simulink model "simulador4"  (Simulink 2.09)
settings: Solver=ode4  StartTime=0.0  StopTime=1  FixedStep=1e-4  MaxStep=0.1  RelTol=1e-3  AbsTol=1e-3
settings Model: SaveTime=off  SaveOutput=off  ConsistencyChecking=off  RTWTemplateMakefile=grt_vc.tmf

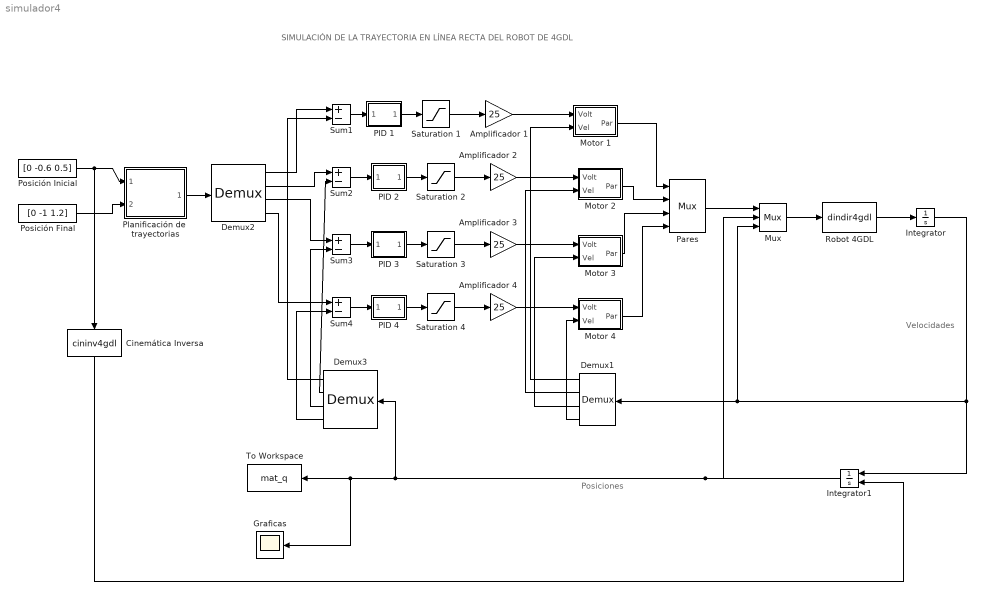
== system simulador4 ==
  note: Velocidades
  note: Posiciones
  note: SIMULACIÓN DE LA TRAYECTORIA EN LÍNEA RECTA DEL ROBOT DE 4GDL
  Amplificador {1..4} (4 alike) : Gain  Gain=25
  Cinemática Inversa : MATLABFcn  Orientation=down  MATLABFcn=cininv4gdl  OutputWidth=4
  Demux1 : Demux  Orientation=left  Outputs=4
  Demux2 : Demux  Outputs=4
  Demux3 : Demux  Orientation=left  Outputs=4
  Graficas : Scope
      settings: TickLabels=on  TimeRange=auto  YMin=-3.25  YMax=1  SaveToWorkspace=off  SaveName=ScopeData
  Integrator : Integrator  ExternalReset=none  InitialConditionSource=internal  InitialCondition=[0 0 0 0]  LimitOutput=off  UpperSaturationLimit=inf  LowerSaturationLimit=-inf  ShowSaturationPort=off  ShowStatePort=off  AbsoluteTolerance=auto
  Integrator1 : Integrator  Orientation=left  ExternalReset=none  InitialConditionSource=external  InitialCondition=[0 0 0 0]  LimitOutput=off  UpperSaturationLimit=inf  LowerSaturationLimit=-inf  ShowSaturationPort=off  ShowStatePort=off  AbsoluteTolerance=auto
  Motor 1 : Subsystem  mask(Motor){R=0.39, L=0.00065, Kt=0.054, Kv=0.054, imax=25.3, red=500}
      mask prompts: R "Resistencia (Ohmios)"; L "Inductancia (Henrios)"; Kt "Kt (Nm/A)"; Kv "Kv (V/rad/s)"; imax "Corriente máxima (Amperios)"; red "Reductor"
  Motor 2 : Subsystem  mask(Motor){R=1.6, L=0.00156, Kt=0.176, Kv=0.176, imax=23.7, red=2}
      mask prompts: R "Resistencia (Ohmios)"; L "Inductancia (Henrios)"; Kt "Kt (Nm/A)"; Kv "Kv (V/rad/s)"; imax "Corriente máxima (Amperios)"; red "Reductor"
  Motor 3 : Subsystem  mask(Motor){R=0.8, L=0.00093, Kt=0.058, Kv=0.058, imax=18.5, red=2}
      mask prompts: R "Resistencia (Ohmios)"; L "Inductancia (Henrios)"; Kt "Kt (N-m)"; Kv "Kv (V/rad/s)"; imax "Corriente máxima (Amperios)"; red "Reductor"
  Motor 4 : Subsystem  mask(Motor){R=6.9, L=0.00128, Kt=0.035, Kv=0.035, imax=3.6, red=500}
      mask prompts: R "Resistencia (Ohmios)"; L "Inductancia (Henrios)"; Kt "Kt (N-m)"; Kv "Kv (V/rad/s)"; imax "Corriente máxima (Amperios)"; red "Reductor"
  Mux : Mux  Inputs=3
  PID 1 : Subsystem  mask(PID Controller){P=90, I=0, D=1.6}
      mask prompts: P "Proportional:"; I "Integral"; D "Derivative:"
      mask help:
      | Enter expressions for proportional, integral, and derivative terms.
      | P+I/s+Ds
      mask Help: This block implements a PID controller where parameters are entered for the Proportional, Integral and Derivative terms. Unmask this block to see how it works. The derivative term is implemented using a true derivative block.
      mask Display: disp('PID')
  PID 2 : Subsystem  mask(PID Controller){P=300, I=0, D=6}
      mask prompts: P "Proportional:"; I "Integral"; D "Derivative:"
      mask help:
      | Enter expressions for proportional, integral, and derivative terms.
      | P+I/s+Ds
      mask Help: This block implements a PID controller where parameters are entered for the Proportional, Integral and Derivative terms. Unmask this block to see how it works. The derivative term is implemented using a true derivative block.
      mask Display: disp('PID')
  PID 3 : Subsystem  mask(PID Controller){P=200, I=0, D=5.7}
      mask prompts: P "Proportional:"; I "Integral"; D "Derivative:"
      mask help:
      | Enter expressions for proportional, integral, and derivative terms.
      | P+I/s+Ds
      mask Help: This block implements a PID controller where parameters are entered for the Proportional, Integral and Derivative terms. Unmask this block to see how it works. The derivative term is implemented using a true derivative block.
      mask Display: disp('PID')
  PID 4 : Subsystem  mask(PID Controller){P=100, I=0, D=0}
      mask prompts: P "Proportional:"; I "Integral"; D "Derivative:"
      mask help:
      | Enter expressions for proportional, integral, and derivative terms.
      | P+I/s+Ds
      mask Help: This block implements a PID controller where parameters are entered for the Proportional, Integral and Derivative terms. Unmask this block to see how it works. The derivative term is implemented using a true derivative block.
      mask Display: disp('PID')
  Pares : Mux  Inputs=4
  Planificación de  trayectorias : Subsystem
      mask Type: Planificación de trayectorias
      mask Display: disp('Planificación')
  Posición Final : Constant  Value=[0 -1 1.2]
  Posición Inicial : Constant  Value=[0 -0.6 0.5]
  Robot 4GDL : MATLABFcn  MATLABFcn=dindir4gdl  OutputWidth=4
  Saturation {1..4} (4 alike) : Saturate  UpperLimit=10  LowerLimit=-10
  Sum{1..4} (4 alike) : Sum  Inputs=+-
  To Workspace : ToWorkspace  VariableName=mat_q  SampleTime=-1
  wires:
  Planificación de  trayectorias/1(Posiciones Articulares) -> Demux2/1
  Cinemática Inversa/1 -> Integrator1/2
  Posición Inicial/1 -> Cinemática Inversa/1, Planificación de  trayectorias/1(Posición Inicial)
  Posición Final/1 -> Planificación de  trayectorias/2(Posición Final)
  Integrator1/1 -> Graficas/1, To Workspace/1, Demux3/1, Mux/2
  Amplificador 3/1 -> Motor 3/1(Volt)
  Amplificador 2/1 -> Motor 2/1(Volt)
  Demux1/2 -> Motor 2/2(Vel)
  Motor 3/1(Par) -> Pares/3
  Motor 2/1(Par) -> Pares/2
  Motor 1/1(Par) -> Pares/1
  Demux1/1 -> Motor 1/2(Vel)
  Demux1/3 -> Motor 3/2(Vel)
  Amplificador 1/1 -> Motor 1/1(Volt)
  Mux/1 -> Robot 4GDL/1
  Pares/1 -> Mux/1
  Demux2/1 -> Sum1/1
  Demux2/2 -> Sum2/1
  Demux2/3 -> Sum3/1
  Demux3/1 -> Sum1/2
  Demux3/2 -> Sum2/2
  Demux3/3 -> Sum3/2
  Sum2/1 -> PID 2/1(In_1)
  Sum3/1 -> PID 3/1(In_1)
  Sum1/1 -> PID 1/1(In_1)
  PID 1/1(Out_1) -> Saturation 1/1
  Saturation 1/1 -> Amplificador 1/1
  PID 2/1(Out_1) -> Saturation 2/1
  Saturation 2/1 -> Amplificador 2/1
  PID 3/1(Out_1) -> Saturation 3/1
  Saturation 3/1 -> Amplificador 3/1
  Integrator/1 -> Integrator1/1, Demux1/1, Mux/3
  Robot 4GDL/1 -> Integrator/1
  Amplificador 4/1 -> Motor 4/1(Volt)
  Sum4/1 -> PID 4/1(In_1)
  PID 4/1(Out_1) -> Saturation 4/1
  Saturation 4/1 -> Amplificador 4/1
  Demux1/4 -> Motor 4/2(Vel)
  Motor 4/1(Par) -> Pares/4
  Demux2/4 -> Sum4/1
  Demux3/4 -> Sum4/2

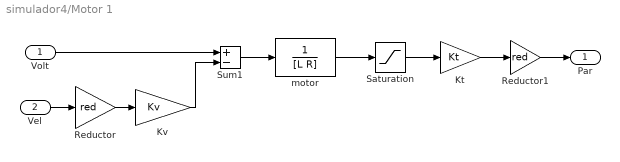
== system simulador4/Motor 1 ==
  Volt : Inport  Port=1  PortWidth=-1  SampleTime=-1
  Vel : Inport  Port=2  PortWidth=-1  SampleTime=-1
  Kt : Gain  Gain=Kt
  Kv : Gain  Gain=Kv
  Reductor : Gain  Gain=red
  Reductor1 : Gain  Gain=red
  Saturation : Saturate  UpperLimit=imax  LowerLimit=-imax
  Sum1 : Sum  Inputs=+-
  motor : TransferFcn  Numerator=[1]  Denominator=[L R]
  Par : Outport  Port=1  InitialOutput=0
  wires:
  Saturation/1 -> Kt/1
  motor/1 -> Saturation/1
  Kt/1 -> Reductor1/1
  Reductor1/1 -> Par/1
  Sum1/1 -> motor/1
  Reductor/1 -> Kv/1
  Kv/1 -> Sum1/2
  Volt/1 -> Sum1/1
  Vel/1 -> Reductor/1

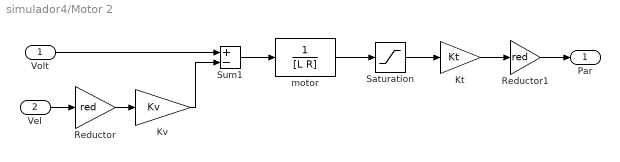
== system simulador4/Motor 2 ==
  Volt : Inport  Port=1  PortWidth=-1  SampleTime=-1
  Vel : Inport  Port=2  PortWidth=-1  SampleTime=-1
  Kt : Gain  Gain=Kt
  Kv : Gain  Gain=Kv
  Reductor : Gain  Gain=red
  Reductor1 : Gain  Gain=red
  Saturation : Saturate  UpperLimit=imax  LowerLimit=-imax
  Sum1 : Sum  Inputs=+-
  motor : TransferFcn  Numerator=[1]  Denominator=[L R]
  Par : Outport  Port=1  InitialOutput=0
  wires:
  Vel/1 -> Reductor/1
  Volt/1 -> Sum1/1
  Kv/1 -> Sum1/2
  Reductor/1 -> Kv/1
  Sum1/1 -> motor/1
  Reductor1/1 -> Par/1
  Kt/1 -> Reductor1/1
  motor/1 -> Saturation/1
  Saturation/1 -> Kt/1

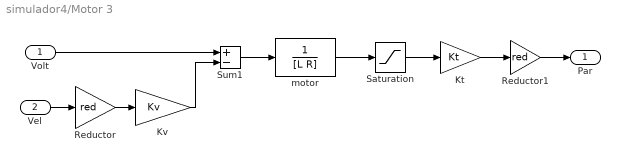
== system simulador4/Motor 3 ==
  Volt : Inport  Port=1  PortWidth=-1  SampleTime=-1
  Vel : Inport  Port=2  PortWidth=-1  SampleTime=-1
  Kt : Gain  Gain=Kt
  Kv : Gain  Gain=Kv
  Reductor : Gain  Gain=red
  Reductor1 : Gain  Gain=red
  Saturation : Saturate  UpperLimit=imax  LowerLimit=-imax
  Sum1 : Sum  Inputs=+-
  motor : TransferFcn  Numerator=[1]  Denominator=[L R]
  Par : Outport  Port=1  InitialOutput=0
  wires:
  Saturation/1 -> Kt/1
  motor/1 -> Saturation/1
  Kt/1 -> Reductor1/1
  Reductor1/1 -> Par/1
  Sum1/1 -> motor/1
  Reductor/1 -> Kv/1
  Kv/1 -> Sum1/2
  Volt/1 -> Sum1/1
  Vel/1 -> Reductor/1

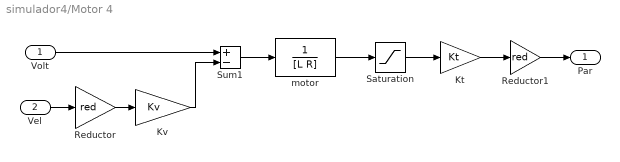
== system simulador4/Motor 4 ==
  Volt : Inport  Port=1  PortWidth=-1  SampleTime=-1
  Vel : Inport  Port=2  PortWidth=-1  SampleTime=-1
  Kt : Gain  Gain=Kt
  Kv : Gain  Gain=Kv
  Reductor : Gain  Gain=red
  Reductor1 : Gain  Gain=red
  Saturation : Saturate  UpperLimit=imax  LowerLimit=-imax
  Sum1 : Sum  Inputs=+-
  motor : TransferFcn  Numerator=[1]  Denominator=[L R]
  Par : Outport  Port=1  InitialOutput=0
  wires:
  Vel/1 -> Reductor/1
  Volt/1 -> Sum1/1
  Kv/1 -> Sum1/2
  Reductor/1 -> Kv/1
  Sum1/1 -> motor/1
  Reductor1/1 -> Par/1
  Kt/1 -> Reductor1/1
  motor/1 -> Saturation/1
  Saturation/1 -> Kt/1

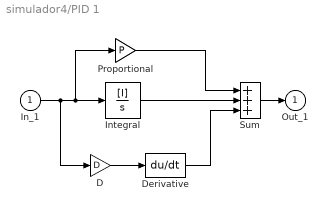
== system simulador4/PID 1 ==
  In_1 : Inport  Port=1  PortWidth=-1  SampleTime=-1
  D : Gain  Gain=D
  Derivative : Derivative
  Integral : TransferFcn  Numerator=[I]  Denominator=[1 0]
  Proportional : Gain  Gain=P
  Sum : Sum  Inputs=+++
  Out_1 : Outport  Port=1  InitialOutput=0
  wires:
  Proportional/1 -> Sum/1
  Integral/1 -> Sum/2
  Derivative/1 -> Sum/3
  In_1/1 -> Proportional/1, Integral/1, D/1
  Sum/1 -> Out_1/1
  D/1 -> Derivative/1

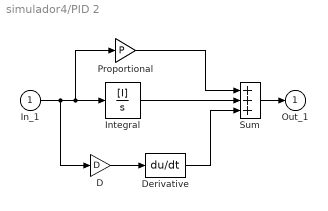
== system simulador4/PID 2 ==
  In_1 : Inport  Port=1  PortWidth=-1  SampleTime=-1
  D : Gain  Gain=D
  Derivative : Derivative
  Integral : TransferFcn  Numerator=[I]  Denominator=[1 0]
  Proportional : Gain  Gain=P
  Sum : Sum  Inputs=+++
  Out_1 : Outport  Port=1  InitialOutput=0
  wires:
  Proportional/1 -> Sum/1
  Integral/1 -> Sum/2
  Derivative/1 -> Sum/3
  In_1/1 -> Proportional/1, Integral/1, D/1
  Sum/1 -> Out_1/1
  D/1 -> Derivative/1

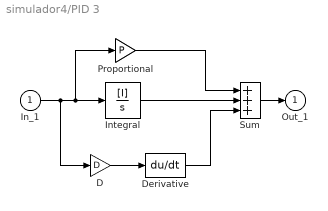
== system simulador4/PID 3 ==
  In_1 : Inport  Port=1  PortWidth=-1  SampleTime=-1
  D : Gain  Gain=D
  Derivative : Derivative
  Integral : TransferFcn  Numerator=[I]  Denominator=[1 0]
  Proportional : Gain  Gain=P
  Sum : Sum  Inputs=+++
  Out_1 : Outport  Port=1  InitialOutput=0
  wires:
  Proportional/1 -> Sum/1
  Integral/1 -> Sum/2
  Derivative/1 -> Sum/3
  In_1/1 -> Proportional/1, Integral/1, D/1
  Sum/1 -> Out_1/1
  D/1 -> Derivative/1

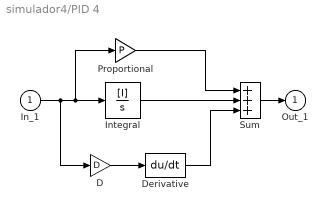
== system simulador4/PID 4 ==
  In_1 : Inport  Port=1  PortWidth=-1  SampleTime=-1
  D : Gain  Gain=D
  Derivative : Derivative
  Integral : TransferFcn  Numerator=[I]  Denominator=[1 0]
  Proportional : Gain  Gain=P
  Sum : Sum  Inputs=+++
  Out_1 : Outport  Port=1  InitialOutput=0
  wires:
  D/1 -> Derivative/1
  Sum/1 -> Out_1/1
  In_1/1 -> D/1, Integral/1, Proportional/1
  Derivative/1 -> Sum/3
  Integral/1 -> Sum/2
  Proportional/1 -> Sum/1

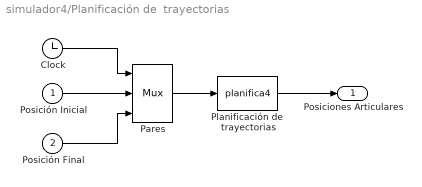
== system simulador4/Planificación de  trayectorias ==
  Posición Inicial : Inport  Port=1  PortWidth=-1  SampleTime=-1
  Posición Final : Inport  Port=2  PortWidth=-1  SampleTime=-1
  Clock : Clock
  Pares : Mux  Inputs=3
  Planificación de  trayectorias : MATLABFcn  MATLABFcn=planifica4  OutputWidth=4
  Posiciones Articulares : Outport  Port=1  InitialOutput=0
  wires:
  Clock/1 -> Pares/1
  Posición Inicial/1 -> Pares/2
  Posición Final/1 -> Pares/3
  Pares/1 -> Planificación de  trayectorias/1
  Planificación de  trayectorias/1 -> Posiciones Articulares/1
